simulink library "sf_bidder"  (R2017b)
settings: Solver=ode45  StartTime=0.0  StopTime=10.0  RelTol=1e-3
settings Model: FPTRunName=Active  ExtModeAutoUpdateStatusClock=off  Creator=The MathWorks, Inc.  LastModifiedBy=The MathWorks, Inc.
settings DataIOCC: LimitDataPoints=on  SaveFormat=Array  SignalLoggingSaveFormat=ModelDataLogs
settings OptimizationCC: BlockReduction=off  BooleanDataType=off  ExpressionDepthLimit=2147483647  LifeSpan=inf
settings DebuggingCC: SaveWithParameterizedLinksMsg=none  UnderspecifiedInitializationDetection=Classic  MergeDetectMultiDrivingBlocksExec=none  SignalResolutionControl=TryResolveAllWithWarning  FcnCallInpInsideContextMsg=warning  StateNameClashWarn=warning  StrictBusMsg=Warning  SFUnexpectedBacktrackingDiag=warning  SFNoUnconditionalDefaultTransitionDiag=warning  SFExecutionAtInitializationDiag=none
settings HardwareCC: ProdBitPerPointer=32  ProdBitPerSizeT=32  ProdBitPerPtrDiffT=32  ProdLargestAtomicFloat=None  ProdIntDivRoundTo=Undefined  ProdEndianess=Unspecified  ProdWordSize=32  ProdHWDeviceType=32-bit Generic  TargetUnknown=on
settings ModelReferenceCC: PropagateSignalLabelsOutOfModel=off
settings CodeAppCC: StateflowObjectComments=on
settings GRTTargetCC: TargetLangStandard=C89/C90 (ANSI)  GeneratePreprocessorConditionals=Disable all  CombineOutputUpdateFcns=off  GRTInterface=on
settings ConfigComp: CovMetricSettings=dcmtr  CovHtmlReporting=on  CovSaveCumulativeToWorkspaceVar=on  CovSaveSingleToWorkspaceVar=on  CovExternalEMLEnable=off

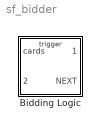
== system sf_bidder ==
  Bidding Logic : Stateflow chart  TreatAsAtomicUnit=on

== stateflow chart sf_bidder/Bidding Logic ==
  state points = count_distribution(suit_count) [function]
    (default) -> (junction 75)
    (junction 75) -> (junction 76) [order 1] : [suit_count < 3] {points = 3-suit_count;}
    (junction 75) -> (junction 74) [order 2] : {points = 0;}
  state bid() [function]
    (default) -> (junction 312)
    (junction 312) -> (junction 314) : {
        | /* Open 1N */
        | aVarTruthTableCondition_1 = (point_count>=16&&point_count<=18);
        | }
    (junction 314) -> (junction 316) : {
        | /* Open 2N */
        | aVarTruthTableCondition_2 = (point_count>=20);
        | }
    (junction 316) -> (junction 318) : {
        | /* Open 2C */
        | aVarTruthTableCondition_3 = (total_points>=22);
        | }
    (junction 318) -> (junction 320) : {
        | /* Opening Count */
        | aVarTruthTableCondition_4 = (total_points>=13);
        | }
    (junction 320) -> (junction 322) : {
        | /* Premptable Count */
        | aVarTruthTableCondition_5 = (point_count>=6);
        | }
    (junction 322) -> (junction 324) : {
        | /* Bid Spades */
        | aVarTruthTableCondition_6 = (spade_count >= 5);
        | }
    (junction 324) -> (junction 326) : {
        | /* Bid Hearts */
        | aVarTruthTableCondition_7 = (heart_count >= 5);
        | }
    (junction 326) -> (junction 328) : {
        | /* Bid Diamonds */
        | aVarTruthTableCondition_8 = (diamond_count >= 4);
        | }
    (junction 328) -> (junction 330) : {
        | /* Preempt Spades */
        | aVarTruthTableCondition_9 = (spade_count >=6);
        | }
    (junction 330) -> (junction 332) : {
        | /* Preempt Hearts */
        | aVarTruthTableCondition_10 = (heart_count >=6);
        | }
    (junction 332) -> (junction 334) : {
        | /* Preempt Diamonds */
        | aVarTruthTableCondition_11 = (diamond_count >= 6);
        | }
    (junction 334) -> (junction 336) : {
        | /* Even Distribution */
        | aVarTruthTableCondition_12 = (distribution_count <= 1);
        | }
    (junction 336) -> (junction 338) [order 1] : [aVarTruthTableCondition_3 && !aVarTruthTableCondition_12]
    (junction 338) -> (junction 340) : {
        | /* Bid 2 */
        | bid_out += 2;
        | }
    (junction 340) -> (junction 342) : {
        | /* 'CLUBS':Bid Clubs */
        | bid_out += club_mask;
        | }
    (junction 336) -> (junction 344) [order 2]
    (junction 344) -> (junction 346) [order 1] : [aVarTruthTableCondition_2 && aVarTruthTableCondition_12]
    (junction 346) -> (junction 348) : {
        | /* Bid 2 */
        | bid_out += 2;
        | }
    (junction 348) -> (junction 350) : {
        | /* 'NO_TRUMP':Bid No Trump */
        | bid_out += no_trump_mask;
        | }
    (junction 344) -> (junction 352) [order 2]
    (junction 352) -> (junction 354) [order 1] : [aVarTruthTableCondition_1 && aVarTruthTableCondition_12]
    (junction 354) -> (junction 356) : {
        | /* Bid 1 */
        | bid_out += 1;
        | }
    (junction 356) -> (junction 358) : {
        | /* 'NO_TRUMP':Bid No Trump */
        | bid_out += no_trump_mask;
        | }
    (junction 352) -> (junction 360) [order 2]
    (junction 360) -> (junction 362) [order 1] : [aVarTruthTableCondition_4 && aVarTruthTableCondition_6]
    (junction 362) -> (junction 364) : {
        | /* Bid 1 */
        | bid_out += 1;
        | }
    (junction 364) -> (junction 366) : {
        | /* 'SPADES':Bid Spades */
        | bid_out += spade_mask;
        | }
    (junction 360) -> (junction 368) [order 2]
    (junction 368) -> (junction 370) [order 1] : [aVarTruthTableCondition_4 && aVarTruthTableCondition_7]
    (junction 370) -> (junction 372) : {
        | /* Bid 1 */
        | bid_out += 1;
        | }
    (junction 372) -> (junction 374) : {
        | /* 'HEARTS':Bid Hearts */
        | bid_out += heart_mask;
        | }
    (junction 368) -> (junction 376) [order 2]
    (junction 376) -> (junction 378) [order 1] : [aVarTruthTableCondition_4 && aVarTruthTableCondition_8]
    (junction 378) -> (junction 380) : {
        | /* Bid 1 */
        | bid_out += 1;
        | }
    (junction 380) -> (junction 382) : {
        | /* 'DIAMONDS':Bid Diamonds */
        | bid_out += diamond_mask;
        | }
    (junction 376) -> (junction 384) [order 2]
    (junction 384) -> (junction 386) [order 1] : [aVarTruthTableCondition_4]
    (junction 386) -> (junction 388) : {
        | /* Bid 1 */
        | bid_out += 1;
        | }
    (junction 388) -> (junction 390) : {
        | /* 'CLUBS':Bid Clubs */
        | bid_out += club_mask;
        | }
    (junction 384) -> (junction 392) [order 2]
    (junction 392) -> (junction 394) [order 1] : [aVarTruthTableCondition_5 && aVarTruthTableCondition_9]
    (junction 394) -> (junction 396) : {
        | /* Bid 2 */
        | bid_out += 2;
        | }
    (junction 396) -> (junction 398) : {
        | /* 'SPADES':Bid Spades */
        | bid_out += spade_mask;
        | }
    (junction 392) -> (junction 400) [order 2]
    (junction 400) -> (junction 402) [order 1] : [aVarTruthTableCondition_5 && aVarTruthTableCondition_10]
    (junction 402) -> (junction 404) : {
        | /* Bid 2 */
        | bid_out += 2;
        | }
    (junction 404) -> (junction 406) : {
        | /* 'HEARTS':Bid Hearts */
        | bid_out += heart_mask;
        | }
    (junction 400) -> (junction 408) [order 2]
    (junction 408) -> (junction 410) [order 1] : [aVarTruthTableCondition_5 && aVarTruthTableCondition_11]
    (junction 410) -> (junction 412) : {
        | /* Bid 2 */
        | bid_out += 2;
        | }
    (junction 412) -> (junction 414) : {
        | /* 'DIAMONDS':Bid Diamonds */
        | bid_out += diamond_mask;
        | }
    (junction 408) -> (junction 416) [order 2]
    (junction 416) -> (junction 418) : /* Default */
    (junction 418) -> (junction 420) : {
        | /* 'PASS':Pass */
        | bid_out = 0;
        | }
  (default) -> (junction 73) [order 1] : DEAL
      | {
      | loop = 0;
      | point_count = 0;
      | distribution_count = 0;
      | club_count = 0;
      | diamond_count = 0;
      | heart_count = 0;
      | spade_count = 0;
      | }
  (junction 80) -> (junction 81)
  (junction 81) -> (junction 73) : {loop++;}
  (junction 79) -> (junction 81) [order 2]
  (junction 82) -> (junction 80)
  (junction 73) -> (junction 79) [order 1] : [loop<13]
      | {
      | club_count += (cards[loop]&club_mask)>0;
      | diamond_count += (cards[loop]&diamond_mask)>0;
      | heart_count += (cards[loop]&heart_mask)>0;
      | spade_count += (cards[loop]&spade_mask)>0;
      | }
  (junction 79) -> (junction 82) [order 1] : [cards[loop] & honor_mask]
      | {point_count+=cards[loop]&card_mask;}
  (junction 73) -> (junction 77) [order 2]
  (default) -> (junction 78) [order 2] : BID
      | {bid_out = 0;}
  (junction 78) -> (junction 84) [order 2] : {NEXT;}
  (junction 78) -> (junction 83) [order 1] : [bid_in == 0]
      | {bid();NEXT;}
  (junction 77) -> (junction 85) : {
      | distribution_count += count_distribution(club_count);
      | distribution_count += count_distribution(diamond_count);
      | distribution_count += count_distribution(heart_count);
      | distribution_count += count_distribution(spade_count);
      | total_points = distribution_count+point_count;
      | }
  data: suit_count function_input double size=1; points function_output double size=1; aVarTruthTableCondition_1 temporary boolean =0; aVarTruthTableCondition_2 temporary boolean =0; aVarTruthTableCondition_3 temporary boolean =0; aVarTruthTableCondition_4 temporary boolean =0; aVarTruthTableCondition_5 temporary boolean =0; aVarTruthTableCondition_6 temporary boolean =0; aVarTruthTableCondition_7 temporary boolean =0; aVarTruthTableCondition_8 temporary boolean =0; aVarTruthTableCondition_9 temporary boolean =0; aVarTruthTableCondition_10 temporary boolean =0; aVarTruthTableCondition_11 temporary boolean =0; aVarTruthTableCondition_12 temporary boolean =0; club_mask constant uint8 size=1 =0x10; diamond_mask constant uint8 size=1 =0x20; heart_mask constant uint8 size=1 =0x40; spade_mask constant uint8 size=1 =0x80; honor_mask constant uint8 size=1 =0x08; point_count local uint8 size=1; club_count local uint8 size=1; diamond_count local uint8 size=1; heart_count local uint8 size=1; spade_count local uint8 size=1; distribution_count local uint8 size=1; total_points local uint8 size=1; loop local uint8 size=1; cards input uint8 size=13; card_mask constant uint8 size=1 =0x07; bid_in input uint8 size=1; bid_out output uint8 size=1; no_trump_mask constant uint8 size=1 =0x08
  data aVarTruthTableCondition_1 settings: description=Open 1N
  data aVarTruthTableCondition_2 settings: description=Open 2N
  data aVarTruthTableCondition_3 settings: description=Open 2C
  data aVarTruthTableCondition_4 settings: description=Opening Count
  data aVarTruthTableCondition_5 settings: description=Premptable Count
  data aVarTruthTableCondition_6 settings: description=Bid Spades
  data aVarTruthTableCondition_7 settings: description=Bid Hearts
  data aVarTruthTableCondition_8 settings: description=Bid Diamonds
  data aVarTruthTableCondition_9 settings: description=Preempt Spades
  data aVarTruthTableCondition_10 settings: description=Preempt Hearts
  data aVarTruthTableCondition_11 settings: description=Preempt Diamonds
  data aVarTruthTableCondition_12 settings: description=Even Distribution
  events: DEAL input EITHER_EDGE_EVENT; BID input EITHER_EDGE_EVENT; NEXT output EITHER_EDGE_EVENT
